simulink model "PID_cart"  (R2024b)
settings: Solver=ode1  StartTime=0.0  StopTime=5  FixedStep=0.002  RelTol=1e-3  EnableMultiTasking=on
PostLoadFcn:
  | qc_set_target_type(getConfigSet(bdroot, 'QUARC Default Target Configuration'));
undefined symbols (not defined in the file): antiwindup_in, den_x, HIL, Kd_in, Ki_in, Kp_in, N_in, num_x, ud_neg, ud_pos, V_sat
libraries: quarc_library x4, simulink x1
settings Model: SimulationMode=external  ExtModeTrigDuration=5000  Creator=pmartin  LastModifiedBy=natha
settings SolverCC: AlgebraicLoopSolver=TrustRegion  PositivePriorityOrder=on
settings DataIOCC: LimitDataPoints=on  SaveFormat=Array  SignalLoggingSaveFormat=ModelDataLogs  ReturnWorkspaceOutputs=off
settings OptimizationCC: ExpressionDepthLimit=2147483647  InitFltsAndDblsToZero=on
settings DebuggingCC: SaveWithParameterizedLinksMsg=none  UnderspecifiedInitializationDetection=Classic  MergeDetectMultiDrivingBlocksExec=none  SolverPrmCheckMsg=warning  MultiTaskDSMMsg=warning  MultiTaskCondExecSysMsg=none  FcnCallInpInsideContextMsg=warning  UnconnectedInputMsg=warning  UnconnectedOutputMsg=warning  UnconnectedLineMsg=warning  StateNameClashWarn=warning  SFUnexpectedBacktrackingDiag=warning  SFNoUnconditionalDefaultTransitionDiag=warning  SFExecutionAtInitializationDiag=none  ArithmeticOperatorsInVariantConditions=warning
settings ModelReferenceCC: PropagateSignalLabelsOutOfModel=off
settings SFSimCC: SimUseLocalCustomCode=off  CustomCodeUndefinedFunction=UseInterfaceOnly
settings RTWCC: RTWUseLocalCustomCode=off  Toolchain=QUARC win64 | nmake (64-bit Windows)  BuildConfiguration=Faster Runs  GPUComputeCapability=3.5
settings CodeAppCC: StateflowObjectComments=on
settings GRTTargetCC: TargetLangStandard=C89/C90 (ANSI)
settings ConfigComp: CovMetricSettings=dw  CovSaveCumulativeToWorkspaceVar=on  CovSaveSingleToWorkspaceVar=on  CovExternalEMLEnable=off

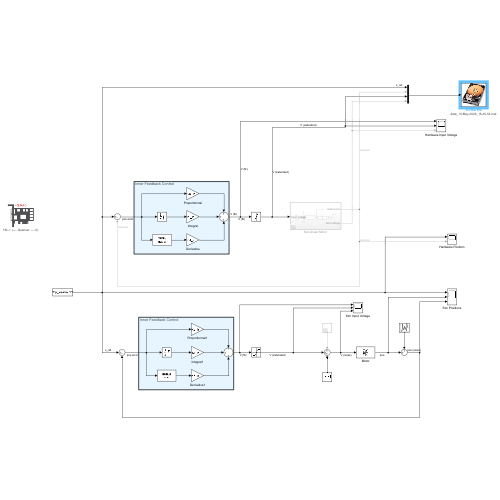
[thumbnail: Simulink's stored preview of the top-level diagram]
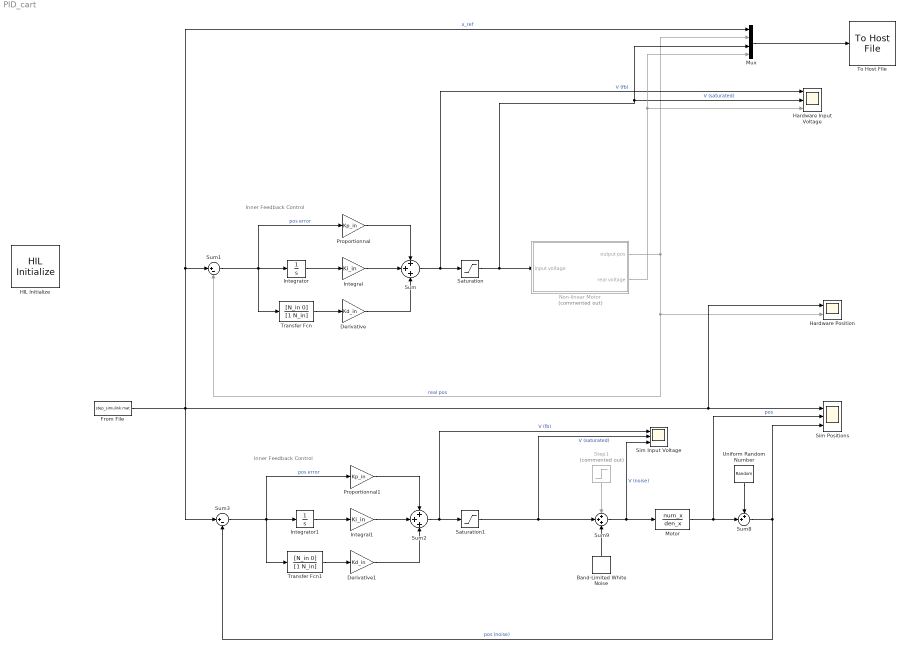
== system PID_cart ==
  note: Inner Feedback Control
  note: Inner Feedback Control
  Band-Limited White Noise : simulink/Sources/Band-Limited White Noise  Cov=[0.000001]  Ts=0.002  seed=[23341]
  Derivative : Gain  Gain=Kd_in
  Derivative1 : Gain  Gain=Kd_in
  From File : FromFile  FileName=step_simulink.mat  SampleTime=0  ExtrapolationBeforeFirstDataPoint=Ground value  ExtrapolationAfterLastDataPoint=Ground value
  HIL Initialize : quarc_library/Data Acquisition/Generic/Configuration/HIL Initialize  object_name=HIL-1  board_type=---- Quanser ----  board_number=0  board_options=d0=digital;d1=digital;led=auto;update_rate=normal  exclusive=off  active=off  hardware_clocks=[0:2]  clock_modes=[]  initial_clock_frequencies=[]  set_clock_params_at_start=off  set_clock_params_at_switch_in=off  set_clock_frequencies_at_start=off  set_clock_frequencies_at_switch_in=off  analog_input_channels=[0:1]  analog_input_configurations=[]  analog_input_maximums=10  analog_input_minimums=-10  set_analog_input_params_at_start=on  set_analog_input_params_at_switch_in=off  analog_output_channels=[0:1]  analog_output_maximums=10  analog_output_minimums=-10  initial_analog_outputs=[0]  final_analog_outputs=[0]  watchdog_analog_outputs=0  set_analog_output_params_at_start=on  set_analog_output_params_at_switch_in=off  set_analog_outputs_at_start=on  set_analog_outputs_at_switch_in=off  set_analog_outputs_at_terminate=on  set_analog_outputs_at_switch_out=off  set_analog_outputs_on_watchdog=off  digital_input_channels=[]  digital_output_channels=[0:7]  digital_output_configuration=[]  initial_digital_outputs=[0]  final_digital_outputs=[0]  watchdog_digital_outputs=[0]  set_digital_output_params_at_start=off  set_digital_output_params_at_switch_in=off  set_digital_outputs_at_start=on  set_digital_outputs_at_switch_in=off  set_digital_outputs_at_terminate=on  set_digital_outputs_at_switch_out=off  set_digital_outputs_on_watchdog=off  encoder_channels=[0:1]  quadrature=[4]  encoder_filter_frequency=[]  initial_encoder_counts=[0]  set_encoder_params_at_start=on  set_encoder_params_at_switch_in=off  set_encoder_counts_at_start=on  set_encoder_counts_at_switch_in=off  pwm_channels=[]  pwm_modes=[0]  pwm_frequency=1/0.020  pwm_configuration=[]  pwm_alignment=[]  pwm_polarity=[]  pwm_leading_deadband=[]  pwm_trailing_deadband=[]  initial_pwm_outputs=[0]  final_pwm_outputs=[0]  watchdog_pwm_outputs=[0]  set_pwm_params_at_start=on  set_pwm_params_at_switch_in=off  set_pwm_outputs_at_start=on  set_pwm_outputs_at_switch_in=off  set_pwm_outputs_at_terminate=on  set_pwm_outputs_at_switch_out=off  set_pwm_outputs_on_watchdog=off  other_output_channels=[]  initial_other_outputs=[]  final_other_outputs=[]  watchdog_other_outputs=[]  set_other_outputs_at_start=off  set_other_outputs_at_switch_in=off  set_other_outputs_at_terminate=off  set_other_outputs_at_switch_out=off  set_other_outputs_on_watchdog=off
  Hardware Input Voltage : Scope  NumInputPorts=3
  Hardware Position : Scope  NumInputPorts=2
  Integral : Gain  Gain=Ki_in
  Integral1 : Gain  Gain=Ki_in
  Integrator : Integrator  LimitOutput=on  UpperSaturationLimit=antiwindup_in  LowerSaturationLimit=-antiwindup_in
  Integrator1 : Integrator  LimitOutput=on  UpperSaturationLimit=antiwindup_in  LowerSaturationLimit=-antiwindup_in
  Motor : TransferFcn  Numerator=num_x  Denominator=den_x
  Mux : Mux
  Non-linear Motor : Subsystem  Commented=on
  Proportionnal : Gain  Gain=Kp_in
  Proportionnal1 : Gain  Gain=Kp_in
  Saturation : Saturate  UpperLimit=V_sat  LowerLimit=-V_sat
  Saturation1 : Saturate  UpperLimit=V_sat  LowerLimit=-V_sat
  Sim Input Voltage : Scope  NumInputPorts=3
  Sim Positions : Scope  NumInputPorts=3
  Step1 : Step  Commented=on  Time=5  SampleTime=0
  Sum : Sum  Inputs=+++
  Sum1 : Sum  Inputs=|+-
  Sum2 : Sum  Inputs=+++
  Sum3 : Sum  Inputs=|+-
  Sum8 : Sum  Inputs=++|
  Sum9 : Sum  Inputs=+++
  To Host File : quarc_library/Sinks/To Host/To Host File  source=Specify via dialog (do not evaluate)  file_name=data_%{date}_%{time}.mat  variable_name=data  decimation=1  sample_time=-1  file_format=MAT-file v.4  options=No header or footer  append=off  final_file_name=data_10-May-2026_18-40-54.mat  encoding=Default  bitrate=0
  Transfer Fcn : TransferFcn  Numerator=[N_in 0]  Denominator=[1 N_in]
  Transfer Fcn1 : TransferFcn  Numerator=[N_in 0]  Denominator=[1 N_in]
  Uniform Random Number : UniformRandomNumber  Minimum=-2.275e-5 * 3  Maximum=2.275e-5 * 3  SampleTime=0.002
  wires:
  Non-linear Motor/1(output pos) -> Mux/2, Sum1/2, Hardware Position/2  "real pos"
  Saturation/1 -> Mux/3, Hardware Input Voltage/2, Non-linear Motor/1(input voltage)  "V (saturated)"
  Sum1/1 -> Transfer Fcn/1, Proportionnal/1, Integrator/1  "pos error"
  Sum/1 -> Saturation/1, Hardware Input Voltage/1  "V (fb)"
  Integrator/1 -> Integral/1
  Proportionnal/1 -> Sum/1
  Integral/1 -> Sum/2
  From File/1 -> Mux/1, Sum1/1, Sum3/1, Hardware Position/1, Sim Positions/1  "x_ref"
  Transfer Fcn/1 -> Derivative/1
  Derivative/1 -> Sum/3
  Mux/1 -> To Host File/1
  Integral1/1 -> Sum2/2
  Sum3/1 -> Transfer Fcn1/1, Proportionnal1/1, Integrator1/1  "pos error"
  Proportionnal1/1 -> Sum2/1
  Derivative1/1 -> Sum2/3
  Integrator1/1 -> Integral1/1
  Transfer Fcn1/1 -> Derivative1/1
  Sum2/1 -> Sim Input Voltage/1, Saturation1/1  "V (fb)"
  Sum9/1 -> Sim Input Voltage/3, Motor/1  "V (noise)"
  Motor/1 -> Sim Positions/2, Sum8/2  "pos"
  Uniform Random Number/1 -> Sum8/1
  Band-Limited White Noise/1 -> Sum9/3
  Step1/1 -> Sum9/1
  Saturation1/1 -> Sim Input Voltage/2, Sum9/2  "V (saturated)"
  Sum8/1 -> Sum3/2, Sim Positions/3  "pos (noise)"
  Non-linear Motor/2(real voltage) -> Mux/4, Hardware Input Voltage/3

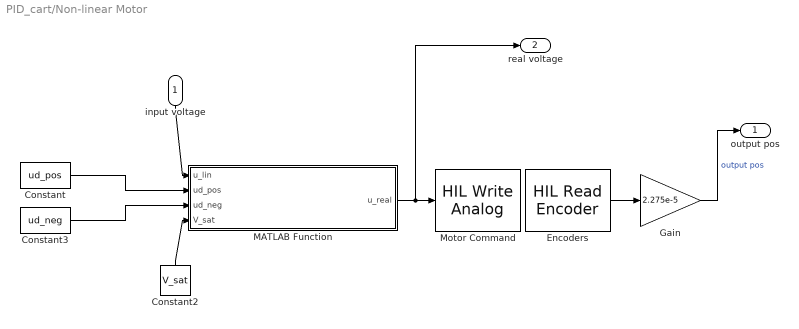
== system PID_cart/Non-linear Motor ==
  input voltage : Inport
  Constant : Constant  Value=ud_pos
  Constant2 : Constant  Value=V_sat
  Constant3 : Constant  Value=ud_neg
  Encoders : quarc_library/Data Acquisition/Generic/Immediate I//O/HIL Read Encoder  object_name=HIL-1  channels=[0]  sample_time=qc_get_step_size  active=on  vector_output=off  data_type_mode=Inherit via back propagation  data_type=double
  Gain : Gain  Gain=2.275e-5
  MATLAB Function : MATLAB Function  TreatAsAtomicUnit=on
  Motor Command : quarc_library/Data Acquisition/Generic/Immediate I//O/HIL Write Analog  object_name=HIL-1  channels=0  sample_time=-1  active=off  vector_input=off
  output pos : Outport
  real voltage : Outport  Port=2
  wires:
  Encoders/1 -> Gain/1
  input voltage/1 -> MATLAB Function/1(u_lin)
  Gain/1 -> output pos/1  "output pos"
  MATLAB Function/1(u_real) -> real voltage/1, Motor Command/1
  Constant/1 -> MATLAB Function/2(ud_pos)
  Constant3/1 -> MATLAB Function/3(ud_neg)
  Constant2/1 -> MATLAB Function/4(V_sat)

== matlab function PID_cart/Non-linear Motor/MATLAB Function ==
  data: u_lin input; u_real output; ud_pos input; ud_neg input; V_sat input
function u_real = non_linear_deadzone(u_lin, ud_pos, ud_neg, V_sat)

epsilon = 0.1;

if u_lin > epsilon
    u_real = u_lin + ud_pos;
    
elseif u_lin < -epsilon
    u_real = u_lin - ud_neg;
    
else
    u_real = 0;
end

if u_real > V_sat
    u_real = V_sat;
elseif u_real < -V_sat
    u_real = -V_sat;
end
